simulink model "REV3"  (R2023b)
settings: Solver=ode8  StartTime=0.0  StopTime=inf  FixedStep=0.0001  RelTol=1e-3
undefined symbols (not defined in the file or in its folder): canChannel
libraries: canmsglib x1, canlib x1
settings Model: DataDictionary=rev3_data.sldd  Creator=rebek  LastModifiedBy=mjmag

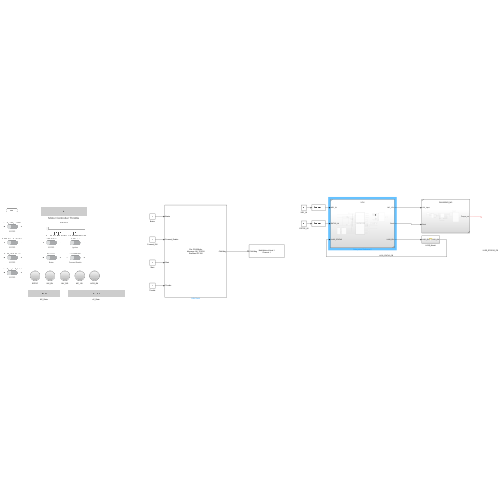
[thumbnail: Simulink's stored preview of the top-level diagram]
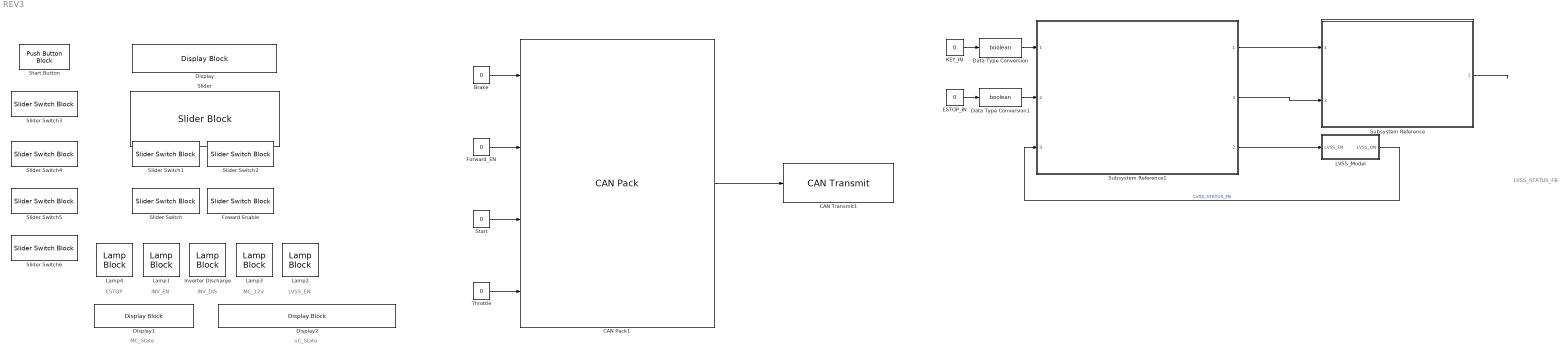
== system REV3 ==
  note: MC_State
  note: LVSS_EN
  note: INV_EN
  note: INV_DIS
  note: LVSS_STATUS_FB
  note: MC_12V
  note: uC_State
  note: ESTOP
  Brake : Constant  Value=0
  CAN Pack1 : canmsglib/CAN Pack  CANdbFile=C:\Users\heyka\MATLAB\Projects\VCU_C\PRJDB.dbc  MsgList=N8_TPDO0  MsgName=N8_TPDO0  MsgIDType=Standard (11-bit identifier)  MsgIdentifier=392  MsgLength=5  Remote=off  ApplyMinMax=off  BusOutput=off  SignalInfo={'Brake','1','16','LE','signed','Standard','0','1','0','0','494967295';'Forward_Enable','0','1','LE','unsigned','Standard','0','1','0','0','494967295';'Start','17','1','LE','unsigned','Standard','0','1','0','-Inf','Inf';'Throttle','18','16','LE','signed','Standard','0','1','0','-32768','32767'}
      settings: LibrarySourceBlock=canlib/CAN Pack  DataFormat=CANdb specified signals
  CAN Transmit1 : canlib/CAN Transmit  BlockHandle=4.0314  Device=MathWorks Virtual 1 (Channel 1)  DeviceMenu=MathWorks Virtual 1 (Channel 1)  ObjConstructor=canChannel('MathWorks', 'Virtual 1', 1)  EnableEventTransmit=off  EnablePeriodicTransmit=off  MessagePeriod=1.000
  Data Type Conversion : DataTypeConversion  OutDataTypeStr=boolean  SaturateOnIntegerOverflow=off  RndMeth=Floor
  Data Type Conversion1 : DataTypeConversion  OutDataTypeStr=boolean  SaturateOnIntegerOverflow=off  RndMeth=Floor
  Display : DisplayBlock  LabelPosition=Hide  Transparency=1
      settings: AttributesFormatString=Motor Controller Throttle
  Display1 : DisplayBlock  LabelPosition=Hide  Transparency=1
  Display2 : DisplayBlock  LabelPosition=Hide  Transparency=1
  ESTOP_IN : Constant  Value=0
  Forward_EN : Constant  Value=0
  Foward Enable : SliderSwitchBlock
      settings: Values={{'Off', 'On'}, [0 1]}
      settings: AttributesFormatString=Forward Enable
  Inverter Discharge : LampBlock  LabelPosition=Hide
  KEY_IN : Constant  Value=0
  LVSS_Model : Subsystem
  Lamp{1..4} (4 alike) : LampBlock  LabelPosition=Hide
  Slider : SliderBlock  ScaleMax=4000
  Slider Switch{,1..6} (7 alike) : SliderSwitchBlock
      settings: Values={{'Off', 'On'}, [0 1]}
      Slider Switch settings: AttributesFormatString=Brake
      Slider Switch1 settings: AttributesFormatString=ESTOP
      Slider Switch2 settings: AttributesFormatString=Ignition
      Slider Switch3 settings: AttributesFormatString=ESTOP
      Slider Switch4 settings: AttributesFormatString=ESTOP
      Slider Switch5 settings: AttributesFormatString=ESTOP
      Slider Switch6 settings: AttributesFormatString=ESTOP
  Start : Constant  Value=0
  Start Button : PushButtonBlock  ButtonText=Start  OffValue=0.000000
  Subsystem Reference : Subsystem  ReferencedSubsystem=PM100DXR_MC
  Subsystem Reference1 : Subsystem  ReferencedSubsystem=VCU
      settings: PortSchema="{\"entries\":[{\"content\":{\"sides\":[{\"content\":{\"connectorIds\":[\"In1\",\"In2\",\"In3\"]},\"type\":\"ConnectorPlacement.EquallySpacedRectSide\",\"uuid\":\"ad158c1f-78bc-4040-9173-78718b9f0641\"},{\"content\":{\"connectorIds\":[\"Out1\",\"Out3\",\"Out2\"],\"side\":\"RIGHT\"},\"type\":\"ConnectorPlacement.EquallySpacedRectSide\",\"uuid\":\"89ea34ac-dfb0-4a0a-b890-23a752478c21\"},{\"content\":{\"side\":\"TOP\"},\"type\":\"ConnectorPlacement.EquallySpacedRectSide\",\"uuid\":\"7119645f-e000-43f4-ab34-6d1534df46a5\"}]},\"type\":\"ConnectorPlacement.EquallySpacedConnector\",\"uuid\":\"7f825ec2-332b-469d-bbcc-991ca31ee6c5\"}],\"packageUris\":[\"http://schema.mathworks.com/mf0/Connector/R2020b\"],\"version\":\"1.0\"}"
  Throttle : Constant  Value=0
  wires:
  KEY_IN/1 -> Data Type Conversion/1
  CAN Pack1/1 -> CAN Transmit1/1
  Forward_EN/1 -> CAN Pack1/2
  Throttle/1 -> CAN Pack1/4
  Start/1 -> CAN Pack1/3
  Brake/1 -> CAN Pack1/1
  Subsystem Reference1/2 -> LVSS_Model/1(LVSS_EN)
  LVSS_Model/1(LVSS_ON) -> Subsystem Reference1/3  "LVSS_STATUS_FB"
  Subsystem Reference1/1 -> Subsystem Reference/1
  Subsystem Reference/1 -> ?
  Subsystem Reference1/3 -> Subsystem Reference/2
  Data Type Conversion/1 -> Subsystem Reference1/1
  ESTOP_IN/1 -> Data Type Conversion1/1
  Data Type Conversion1/1 -> Subsystem Reference1/2

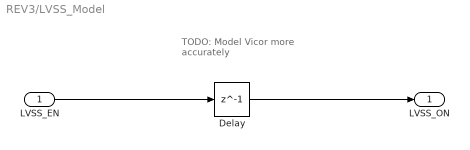
== system REV3/LVSS_Model ==
  note: TODO: Model Vicor more accurately
  LVSS_EN : Inport
  Delay : Delay  DelayLength=1
  LVSS_ON : Outport
  wires:
  LVSS_EN/1 -> Delay/1
  Delay/1 -> LVSS_ON/1
